simulink model "QDPSK"  (R2018b)
settings: Solver=FixedStepDiscrete  StartTime=0.0  StopTime=(1/Rb)*CantBit  RelTol=1e-3
values from neighbouring files (symbols this model uses):
  Eb = EbPerf    [BDPSK.m]    (also in Codigo8DPSK.m; CodigoQDPSK.m)
  Es = 1*Eb    [BDPSK.m]    (also in Codigo8DPSK.m = 3*Eb; CodigoQDPSK.m = 2*Eb)
  Fp = 10*Rb    [BDPSK.m]    (also in Codigo8DPSK.m; CodigoQDPSK.m)
  Fs = FsPerf    [Codigo8DPSK.m]    (also in CodigoQDPSK.m)
  Rb = RbPerf    [BDPSK.m]    (also in Codigo8DPSK.m; CodigoQDPSK.m)
  Rs = Rb/1    [BDPSK.m]    (also in Codigo8DPSK.m = Rb/3; CodigoQDPSK.m = Rb/2)
libraries: commfilt2 x2, commdigbbndpm3 x2, commchan3 x1, commrandsrc2 x1, commutil2 x1
settings Model: Creator=lukit  LastModifiedBy=lukit

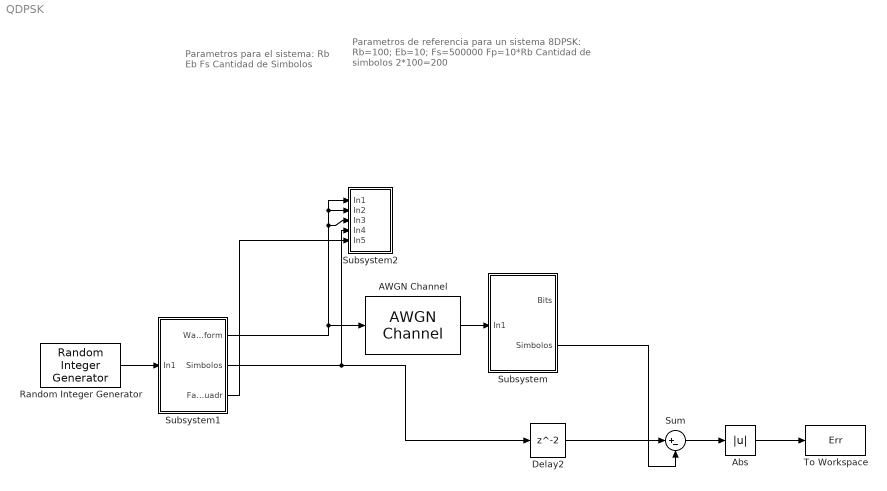
== system QDPSK ==
  note: Parametros de referencia para un sistema 8DPSK:
      | Rb=100;
      | Eb=10;
      | Fs=500000
      | Fp=10*Rb
      | Cantidad de simbolos 2*100=200
  note: Parametros para el sistema:
      | Rb
      | Eb
      | Fs
      | Cantidad de Simbolos
  AWGN Channel : commchan3/AWGN Channel  InputProcessing=Columns as channels (frame based)  seed=67  noiseMode="Signal to noise ratio  (Es/No)"  EbNodB=10  EsNodB=EsNo  SNRdB=10  bitsPerSym=3  Ps=Eb/(1/Rb)  Tsym=(1/Rb)*3  variance=25
  Abs : Abs
  Delay2 : Delay  InitialCondition=0
  Random Integer Generator : commrandsrc2/Random Integer Generator  mul=2  seed=randseed  Ts=1/Rb  frameBased=off  sampPerFrame=1  orient=off  outDataType=double
  Subsystem : Subsystem
  Subsystem1 : Subsystem
  Subsystem2 : Subsystem
  Sum : Sum  Inputs=|+-
  To Workspace : ToWorkspace  VariableName=Err  SampleTime=1/Rs
      settings: Save2DSignal=2-D array (concatenate along first dimension)
  wires:
  Random Integer Generator/1 -> Subsystem1/1(In1)
  Subsystem1/2(Simbolos) -> Subsystem2/4(In4), Delay2/1
  Subsystem1/1(Waveform) -> Subsystem2/3(In3), Subsystem2/1(In1), Subsystem2/2(In2), AWGN Channel/1
  Delay2/1 -> Sum/1
  Subsystem/2(Simbolos) -> Sum/2
  Sum/1 -> Abs/1
  Abs/1 -> To Workspace/1
  Subsystem1/3(Fas/Cuadr) -> Subsystem2/5(In5)
  AWGN Channel/1 -> Subsystem/1(In1)

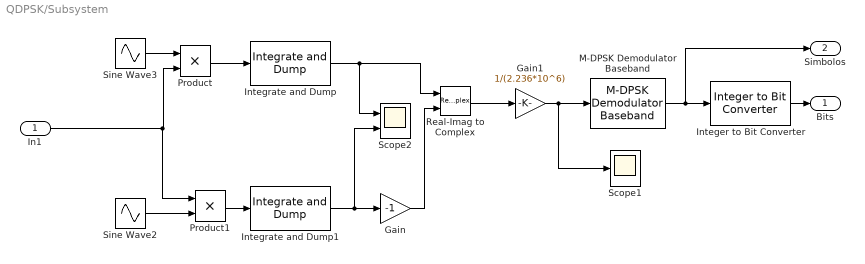
== system QDPSK/Subsystem ==
  In1 : Inport
  Gain : Gain  Gain=-1
  Gain1 : Gain  Gain=1/(2.236*10^6)
  Integer to Bit Converter : commutil2/Integer to Bit Converter  nbits=2  signedInputValues=Unsigned  bitOrder=MSB first  outDtype=boolean
  Integrate and Dump : commfilt2/Integrate and Dump  obssamples=(1/Rs)*Fs  offsetsamples=0  nodump=off  roundingMode=Floor  overflowMode=off  outputDataTypeStr=Inherit: Same as accumulator  outputLastDataTypeStr=Inherit: Same as accumulator
      settings: SourceProductName=Communications Toolbox
  Integrate and Dump1 : commfilt2/Integrate and Dump  obssamples=(1/Rs)*Fs  offsetsamples=0  nodump=off  roundingMode=Floor  overflowMode=off  outputDataTypeStr=Inherit: Same as accumulator  outputLastDataTypeStr=Inherit: Same as accumulator
      settings: SourceProductName=Communications Toolbox
  M-DPSK Demodulator Baseband : commdigbbndpm3/M-DPSK Demodulator Baseband  M=4  OutType=Integer  Dec=Gray  Ph=0  outDtype1=Inherit via internal rule  outDtype2=Inherit via internal rule
      settings: SourceProductName=Communications System Toolbox  SourceProductBaseCode=CM
  Product : Product
  Product1 : Product
  Real-Imag to Complex : RealImagToComplex
  Scope1 : Scope
  Scope2 : Scope  NumInputPorts=2
  Sine Wave2 : Sin  Amplitude=sqrt(2/(1/Rs))  Frequency=2*pi*Fp  SampleTime=1/Fs
  Sine Wave3 : Sin  Amplitude=sqrt(2/(1/Rs))  Frequency=2*pi*Fp  Phase=pi/2  SampleTime=1/Fs
  Bits : Outport
  Simbolos : Outport  Port=2
  wires:
  Gain1/1 -> Scope1/1, M-DPSK Demodulator Baseband/1
  Gain/1 -> Real-Imag to Complex/2
  Product/1 -> Integrate and Dump/1
  In1/1 -> Product1/1, Product/2
  Integrate and Dump1/1 -> Scope2/2, Gain/1
  Integrate and Dump/1 -> Scope2/1, Real-Imag to Complex/1
  Product1/1 -> Integrate and Dump1/1
  M-DPSK Demodulator Baseband/1 -> Simbolos/1, Integer to Bit Converter/1
  Real-Imag to Complex/1 -> Gain1/1
  Sine Wave3/1 -> Product/1
  Sine Wave2/1 -> Product1/2
  Integer to Bit Converter/1 -> Bits/1

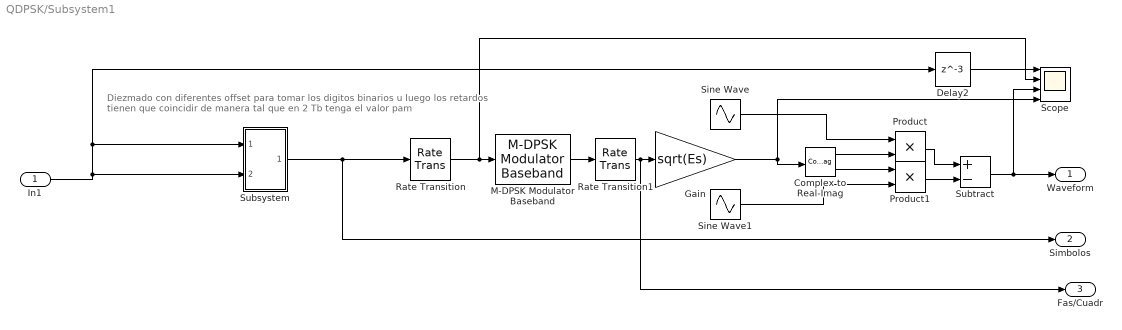
== system QDPSK/Subsystem1 ==
  note: Diezmado con diferentes offset para tomar los digitos binarios u luego los retardos
      | tienen que coincidir de manera tal que en 2 Tb tenga el valor pam
  In1 : Inport
  Complex to Real-Imag : ComplexToRealImag
  Delay2 : Delay  DelayLength=3  InitialCondition=0
  Gain : Gain  Gain=sqrt(Es)
  M-DPSK Modulator Baseband : commdigbbndpm3/M-DPSK Modulator Baseband  M=4  InType=Integer  Enc=Gray  Ph=0  outDtype=double
      settings: SourceProductName=Communications System Toolbox  SourceProductBaseCode=CM
  Product : Product
  Product1 : Product
  Rate Transition : RateTransition  OutPortSampleTime=1/Rs
  Rate Transition1 : RateTransition  OutPortSampleTime=1/Fs
  Scope : Scope  NumInputPorts=4
  Sine Wave : Sin  Amplitude=sqrt(2/(1/Rs))  Frequency=2*pi*Fp  Phase=pi/2  SampleTime=1/Fs
  Sine Wave1 : Sin  Amplitude=sqrt(2/(1/Rs))  Frequency=2*pi*Fp  SampleTime=1/Fs
  Subsystem : Subsystem
  Subtract : Sum  Inputs=+-
  Waveform : Outport
  Simbolos : Outport  Port=2
  Fas/Cuadr : Outport  Port=3
  wires:
  Complex to Real-Imag/1 -> Product/2
  Complex to Real-Imag/2 -> Product1/1
  Gain/1 -> Complex to Real-Imag/1, Scope/4
  Subtract/1 -> Waveform/1, Scope/3
  Sine Wave1/1 -> Product1/2
  In1/1 -> Subsystem/2(In2), Delay2/1, Subsystem/1(In1)
  Rate Transition/1 -> M-DPSK Modulator Baseband/1, Scope/2
  Delay2/1 -> Scope/1
  Product1/1 -> Subtract/2
  Product/1 -> Subtract/1
  Sine Wave/1 -> Product/1
  Rate Transition1/1 -> Fas/Cuadr/1, Gain/1
  M-DPSK Modulator Baseband/1 -> Rate Transition1/1
  Subsystem/1(Out1) -> Simbolos/1, Rate Transition/1

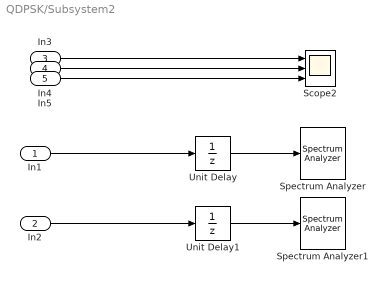
== system QDPSK/Subsystem2 ==
  In1 : Inport
  In2 : Inport  Port=2
  In3 : Inport  Port=3
  In4 : Inport  Port=4
  In5 : Inport  Port=5
  Scope2 : Scope  NumInputPorts=3
  Spectrum Analyzer : SpectrumAnalyzer
  Spectrum Analyzer1 : SpectrumAnalyzer
  Unit Delay : UnitDelay  SampleTime=1/Fs
  Unit Delay1 : UnitDelay  SampleTime=1/Fs
  wires:
  Unit Delay/1 -> Spectrum Analyzer/1
  In1/1 -> Unit Delay/1
  In2/1 -> Unit Delay1/1
  Unit Delay1/1 -> Spectrum Analyzer1/1
  In3/1 -> Scope2/1
  In4/1 -> Scope2/2
  In5/1 -> Scope2/3

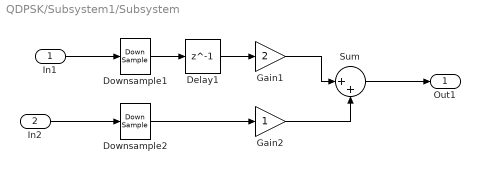
== system QDPSK/Subsystem1/Subsystem ==
  In1 : Inport
  In2 : Inport  Port=2
  Delay1 : Delay  DelayLength=1  InitialCondition=0
  Downsample1 : DownSample  RateOptions=Allow multirate processing
  Downsample2 : DownSample  phase=1  RateOptions=Allow multirate processing
  Gain1 : Gain  Gain=2
  Gain2 : Gain
  Sum : Sum  Inputs=|++
  Out1 : Outport
  wires:
  Gain1/1 -> Sum/1
  Downsample2/1 -> Gain2/1
  Sum/1 -> Out1/1
  Downsample1/1 -> Delay1/1
  Delay1/1 -> Gain1/1
  Gain2/1 -> Sum/2
  In2/1 -> Downsample2/1
  In1/1 -> Downsample1/1
